simulink model "chernobyl_sim"  (R2022b)
settings: Solver=VariableStepAuto  StartTime=0.0  StopTime=10.0  RelTol=1e-3
values from neighbouring files (symbols this model uses):
  k_c137 = log(2)/30*segundosporanyo    [chernobyl.m]
  k_y131 = log(2)/8*segundospordia    [chernobyl.m]
  toneladaKg = 1000    [chernobyl.m]
settings Model: Creator=Fran  LastModifiedBy=Fran

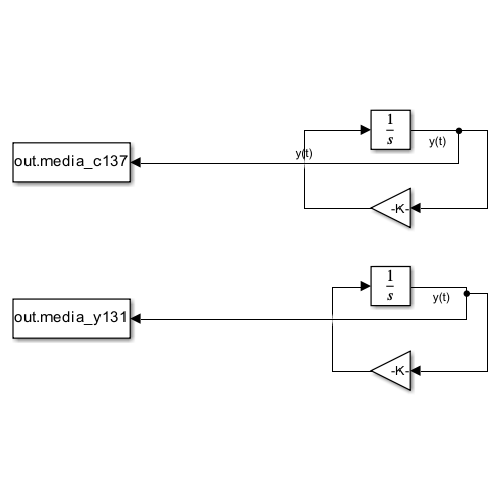
[thumbnail: Simulink's stored preview of the top-level diagram]
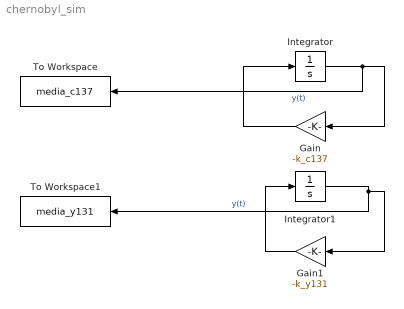
== system chernobyl_sim ==
  Gain : Gain  Gain=-k_c137
  Gain1 : Gain  Gain=-k_y131
  Integrator : Integrator  InitialCondition=1000
  Integrator1 : Integrator  InitialCondition=100*toneladaKg
  To Workspace : ToWorkspace  VariableName=media_c137  SampleTime=-1
  To Workspace1 : ToWorkspace  VariableName=media_y131  SampleTime=-1
  wires:
  Gain/1 -> Integrator/1
  Integrator/1 -> To Workspace/1, Gain/1  "y(t)"
  Gain1/1 -> Integrator1/1
  Integrator1/1 -> To Workspace1/1, Gain1/1  "y(t)"
